simulink model "cic_filter_test_bitgrowthissue"  (Simulink 7.4)
settings: Solver=ode45  StartTime=0.0  StopTime=10000  RelTol=1e-3
libraries: xbsIndex_r4 x288, simulink x2, xrbsComm_r4 x1, xps_library x1
(part 2 of 3)

== system cic_filter_test_bitgrowthissue/myCIC/stage2 ==
  in1 : Inport
  in2 : Inport  Port=2
  sync : Inport  Port=3
  final_adder1 : xbsIndex_r4/AddSub  mode=Addition  use_carryin=off  use_carryout=off  en=off  latency=1  precision=Full  arith_type=Unsigned  n_bits=16  bin_pt=14  quantization=Truncate  overflow=Wrap  dbl_ovrd=off  use_behavioral_HDL=off  hw_selection=Fabric  pipelined=off  block_type=addsub
  polynomial0 : Subsystem
  polynomial1 : Subsystem
  sync_delay : xbsIndex_r4/Delay  en=off  latency=1  dbl_ovrd=off  reg_retiming=off  block_type=delay
      settings: block_version=11.4
  out1 : Outport
  sync_out : Outport  Port=2
  wires:
  sync/1 -> polynomial1/2(sync), polynomial0/2(sync)
  polynomial0/3(sync_out) -> sync_delay/1  "sync_poly"
  final_adder1/1 -> out1/1
  polynomial0/2(out_even) -> final_adder1/1  "poly_out0_even"
  in1/1 -> polynomial0/1(in)
  in2/1 -> polynomial1/1(in)
  polynomial1/1(out_odd) -> final_adder1/2  "poly_out1_odd"
  sync_delay/1 -> sync_out/1

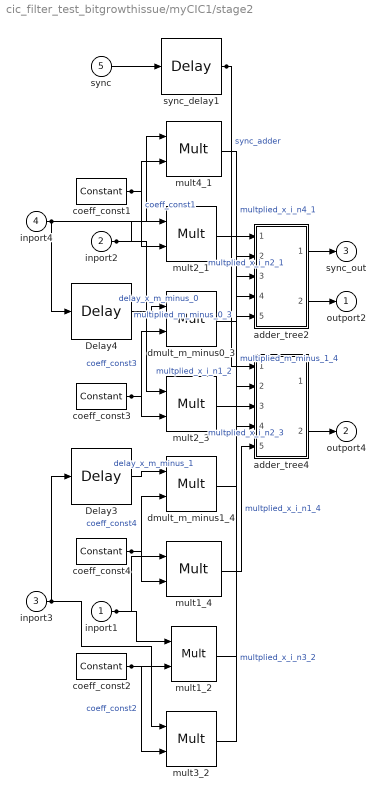
== system cic_filter_test_bitgrowthissue/myCIC1/stage2 ==
  inport1 : Inport
  inport2 : Inport  Port=2
  inport3 : Inport  Port=3
  inport4 : Inport  Port=4
  sync : Inport  Port=5
  Delay3 : xbsIndex_r4/Delay  en=off  latency=1  dbl_ovrd=off  reg_retiming=off  block_type=delay
      settings: block_version=11.4
  Delay4 : xbsIndex_r4/Delay  en=off  latency=1  dbl_ovrd=off  reg_retiming=off  block_type=delay
      settings: block_version=11.4
  adder_tree2 : Subsystem
  adder_tree4 : Subsystem
  coeff_const1 : xbsIndex_r4/Constant  arith_type=Unsigned  const=1  n_bits=3  bin_pt=0  explicit_period=off  period=1  equ=P=C  opselect=C  inp2=PCIN>>17  opr=+  inp1=P  carry=CIN  dbl_ovrd=off  block_type=constant
      settings: block_version=11.4
  coeff_const2 : xbsIndex_r4/Constant  arith_type=Unsigned  const=3  n_bits=3  bin_pt=0  explicit_period=off  period=1  equ=P=C  opselect=C  inp2=PCIN>>17  opr=+  inp1=P  carry=CIN  dbl_ovrd=off  block_type=constant
      settings: block_version=11.4
  coeff_const3 : xbsIndex_r4/Constant  arith_type=Unsigned  const=3  n_bits=3  bin_pt=0  explicit_period=off  period=1  equ=P=C  opselect=C  inp2=PCIN>>17  opr=+  inp1=P  carry=CIN  dbl_ovrd=off  block_type=constant
      settings: block_version=11.4
  coeff_const4 : xbsIndex_r4/Constant  arith_type=Unsigned  const=1  n_bits=3  bin_pt=0  explicit_period=off  period=1  equ=P=C  opselect=C  inp2=PCIN>>17  opr=+  inp1=P  carry=CIN  dbl_ovrd=off  block_type=constant
      settings: block_version=11.4
  dmult_m_minus0_3 : xbsIndex_r4/Mult  precision=Full  arith_type="Signed  (2's comp)"  n_bits=16  bin_pt=14  quantization=Truncate  overflow=Wrap  en=off  latency=2  dbl_ovrd=off  use_behavioral_HDL=off  opt=Speed  use_embedded=on  optimum_pipeline=off  pipeline=on  use_rpm=on  placement_style=Triangular  block_type=mult
      settings: block_version=11.4
  dmult_m_minus1_4 : xbsIndex_r4/Mult  precision=Full  arith_type="Signed  (2's comp)"  n_bits=16  bin_pt=14  quantization=Truncate  overflow=Wrap  en=off  latency=2  dbl_ovrd=off  use_behavioral_HDL=off  opt=Speed  use_embedded=on  optimum_pipeline=off  pipeline=on  use_rpm=on  placement_style=Triangular  block_type=mult
      settings: block_version=11.4
  mult1_2 : xbsIndex_r4/Mult  precision=Full  arith_type="Signed  (2's comp)"  n_bits=16  bin_pt=14  quantization=Truncate  overflow=Wrap  en=off  latency=2  dbl_ovrd=off  use_behavioral_HDL=off  opt=Speed  use_embedded=on  optimum_pipeline=off  pipeline=on  use_rpm=on  placement_style=Triangular  block_type=mult
      settings: block_version=11.4
  mult1_4 : xbsIndex_r4/Mult  precision=Full  arith_type="Signed  (2's comp)"  n_bits=16  bin_pt=14  quantization=Truncate  overflow=Wrap  en=off  latency=2  dbl_ovrd=off  use_behavioral_HDL=off  opt=Speed  use_embedded=on  optimum_pipeline=off  pipeline=on  use_rpm=on  placement_style=Triangular  block_type=mult
      settings: block_version=11.4
  mult2_1 : xbsIndex_r4/Mult  precision=Full  arith_type="Signed  (2's comp)"  n_bits=16  bin_pt=14  quantization=Truncate  overflow=Wrap  en=off  latency=2  dbl_ovrd=off  use_behavioral_HDL=off  opt=Speed  use_embedded=on  optimum_pipeline=off  pipeline=on  use_rpm=on  placement_style=Triangular  block_type=mult
      settings: block_version=11.4
  mult2_3 : xbsIndex_r4/Mult  precision=Full  arith_type="Signed  (2's comp)"  n_bits=16  bin_pt=14  quantization=Truncate  overflow=Wrap  en=off  latency=2  dbl_ovrd=off  use_behavioral_HDL=off  opt=Speed  use_embedded=on  optimum_pipeline=off  pipeline=on  use_rpm=on  placement_style=Triangular  block_type=mult
      settings: block_version=11.4
  mult3_2 : xbsIndex_r4/Mult  precision=Full  arith_type="Signed  (2's comp)"  n_bits=16  bin_pt=14  quantization=Truncate  overflow=Wrap  en=off  latency=2  dbl_ovrd=off  use_behavioral_HDL=off  opt=Speed  use_embedded=on  optimum_pipeline=off  pipeline=on  use_rpm=on  placement_style=Triangular  block_type=mult
      settings: block_version=11.4
  mult4_1 : xbsIndex_r4/Mult  precision=Full  arith_type="Signed  (2's comp)"  n_bits=16  bin_pt=14  quantization=Truncate  overflow=Wrap  en=off  latency=2  dbl_ovrd=off  use_behavioral_HDL=off  opt=Speed  use_embedded=on  optimum_pipeline=off  pipeline=on  use_rpm=on  placement_style=Triangular  block_type=mult
      settings: block_version=11.4
  sync_delay1 : xbsIndex_r4/Delay  en=off  latency=2  dbl_ovrd=off  reg_retiming=off  block_type=delay
      settings: block_version=11.4
  outport2 : Outport
  outport4 : Outport  Port=2
  sync_out : Outport  Port=3
  wires:
  inport1/1 -> mult1_2/1, mult1_4/1
  coeff_const4/1 -> mult1_4/2, dmult_m_minus1_4/2  "coeff_const4"
  inport2/1 -> mult2_1/1, mult2_3/1
  coeff_const3/1 -> mult2_3/2, dmult_m_minus0_3/2  "coeff_const3"
  inport3/1 -> mult3_2/1, Delay3/1
  coeff_const2/1 -> mult1_2/2, mult3_2/2  "coeff_const2"
  inport4/1 -> Delay4/1, mult4_1/1
  coeff_const1/1 -> mult4_1/2, mult2_1/2  "coeff_const1"
  sync_delay1/1 -> adder_tree4/1(sync), adder_tree2/1(sync)  "sync_adder"
  mult1_4/1 -> adder_tree4/5(din_4)  "multplied_x_i_n1_4"
  mult3_2/1 -> adder_tree4/3(din_2)  "multplied_x_i_n3_2"
  adder_tree2/2(dout) -> outport2/1
  dmult_m_minus1_4/1 -> adder_tree2/5(din_4)  "multiplied_m_minus_1_4"
  mult1_2/1 -> adder_tree2/3(din_2)  "multplied_x_i_n1_2"
  sync/1 -> sync_delay1/1
  Delay4/1 -> dmult_m_minus0_3/1  "delay_x_m_minus_0"
  Delay3/1 -> dmult_m_minus1_4/1  "delay_x_m_minus_1"
  mult2_1/1 -> adder_tree2/2(din_1)  "multplied_x_i_n2_1"
  dmult_m_minus0_3/1 -> adder_tree2/4(din_3)  "multiplied_m_minus_0_3"
  adder_tree2/1(sync_out) -> sync_out/1
  mult4_1/1 -> adder_tree4/2(din_1)  "multplied_x_i_n4_1"
  mult2_3/1 -> adder_tree4/4(din_3)  "multplied_x_i_n2_3"
  adder_tree4/2(dout) -> outport4/1

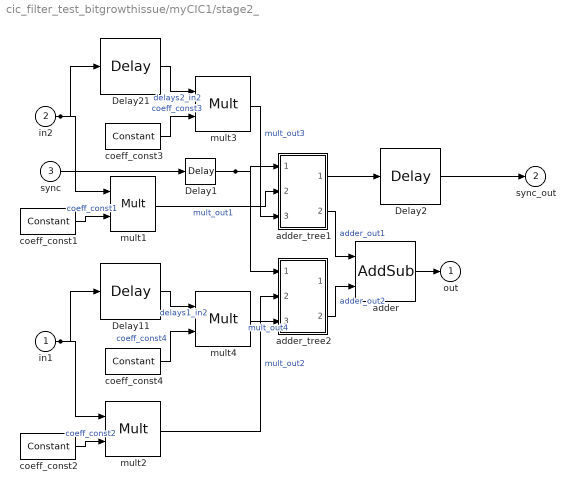
== system cic_filter_test_bitgrowthissue/myCIC1/stage2_ ==
  in1 : Inport
  in2 : Inport  Port=2
  sync : Inport  Port=3
  Delay1 : xbsIndex_r4/Delay  en=off  latency=2  dbl_ovrd=off  reg_retiming=off  block_type=delay
      settings: block_version=11.4
  Delay11 : xbsIndex_r4/Delay  en=off  latency=1  dbl_ovrd=off  reg_retiming=off  block_type=delay
      settings: block_version=11.4
  Delay2 : xbsIndex_r4/Delay  en=off  latency=1  dbl_ovrd=off  reg_retiming=off  block_type=delay
      settings: block_version=11.4
  Delay21 : xbsIndex_r4/Delay  en=off  latency=1  dbl_ovrd=off  reg_retiming=off  block_type=delay
      settings: block_version=11.4
  adder : xbsIndex_r4/AddSub  mode=Addition  use_carryin=off  use_carryout=off  en=off  latency=1  precision=Full  arith_type=Unsigned  n_bits=16  bin_pt=14  quantization=Truncate  overflow=Wrap  dbl_ovrd=off  use_behavioral_HDL=off  hw_selection=Fabric  pipelined=off  block_type=addsub
  adder_tree1 : Subsystem
  adder_tree2 : Subsystem
  coeff_const1 : xbsIndex_r4/Constant  arith_type=Unsigned  const=1  n_bits=3  bin_pt=0  explicit_period=off  period=1  equ=P=C  opselect=C  inp2=PCIN>>17  opr=+  inp1=P  carry=CIN  dbl_ovrd=off  block_type=constant
      settings: block_version=11.4
  coeff_const2 : xbsIndex_r4/Constant  arith_type=Unsigned  const=3  n_bits=3  bin_pt=0  explicit_period=off  period=1  equ=P=C  opselect=C  inp2=PCIN>>17  opr=+  inp1=P  carry=CIN  dbl_ovrd=off  block_type=constant
      settings: block_version=11.4
  coeff_const3 : xbsIndex_r4/Constant  arith_type=Unsigned  const=3  n_bits=3  bin_pt=0  explicit_period=off  period=1  equ=P=C  opselect=C  inp2=PCIN>>17  opr=+  inp1=P  carry=CIN  dbl_ovrd=off  block_type=constant
      settings: block_version=11.4
  coeff_const4 : xbsIndex_r4/Constant  arith_type=Unsigned  const=1  n_bits=3  bin_pt=0  explicit_period=off  period=1  equ=P=C  opselect=C  inp2=PCIN>>17  opr=+  inp1=P  carry=CIN  dbl_ovrd=off  block_type=constant
      settings: block_version=11.4
  mult{1..4} (4 alike) : xbsIndex_r4/Mult  precision=Full  arith_type="Signed  (2's comp)"  n_bits=16  bin_pt=14  quantization=Truncate  overflow=Wrap  en=off  latency=2  dbl_ovrd=off  use_behavioral_HDL=off  opt=Speed  use_embedded=on  optimum_pipeline=off  pipeline=on  use_rpm=on  placement_style=Triangular  block_type=mult
      settings: block_version=11.4
  out : Outport
  sync_out : Outport  Port=2
  wires:
  in2/1 -> mult1/1, Delay21/1
  in1/1 -> Delay11/1, mult2/1
  sync/1 -> Delay1/1
  adder_tree2/2(dout) -> adder/2  "adder_out2"
  mult2/1 -> adder_tree2/2(din_1)  "mult_out2"
  mult3/1 -> adder_tree1/3(din_2)  "mult_out3"
  coeff_const4/1 -> mult4/2  "coeff_const4"
  Delay21/1 -> mult3/1  "delays2_in2"
  coeff_const2/1 -> mult2/2  "coeff_const2"
  coeff_const1/1 -> mult1/2  "coeff_const1"
  coeff_const3/1 -> mult3/2  "coeff_const3"
  Delay11/1 -> mult4/1  "delays1_in2"
  mult1/1 -> adder_tree1/2(din_1)  "mult_out1"
  adder_tree1/1(sync_out) -> Delay2/1
  mult4/1 -> adder_tree2/3(din_2)  "mult_out4"
  adder_tree1/2(dout) -> adder/1  "adder_out1"
  adder/1 -> out/1
  Delay1/1 -> adder_tree1/1(sync), adder_tree2/1(sync)
  Delay2/1 -> sync_out/1

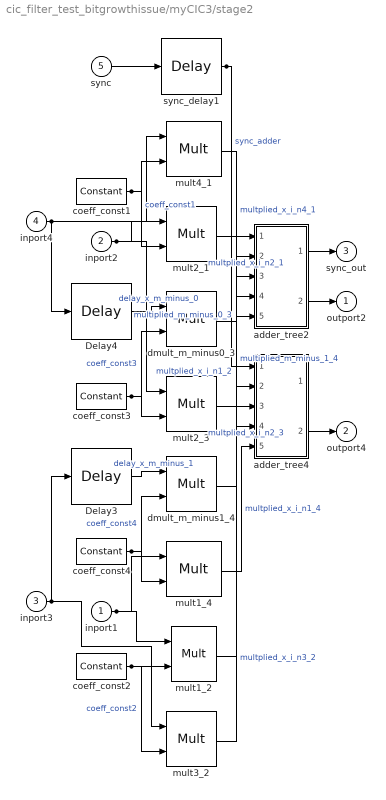
== system cic_filter_test_bitgrowthissue/myCIC3/stage2 ==
  inport1 : Inport
  inport2 : Inport  Port=2
  inport3 : Inport  Port=3
  inport4 : Inport  Port=4
  sync : Inport  Port=5
  Delay3 : xbsIndex_r4/Delay  en=off  latency=1  dbl_ovrd=off  reg_retiming=off  block_type=delay
      settings: block_version=11.4
  Delay4 : xbsIndex_r4/Delay  en=off  latency=1  dbl_ovrd=off  reg_retiming=off  block_type=delay
      settings: block_version=11.4
  adder_tree2 : Subsystem
  adder_tree4 : Subsystem
  coeff_const1 : xbsIndex_r4/Constant  arith_type=Unsigned  const=1  n_bits=3  bin_pt=0  explicit_period=off  period=1  equ=P=C  opselect=C  inp2=PCIN>>17  opr=+  inp1=P  carry=CIN  dbl_ovrd=off  block_type=constant
      settings: block_version=11.4
  coeff_const2 : xbsIndex_r4/Constant  arith_type=Unsigned  const=3  n_bits=3  bin_pt=0  explicit_period=off  period=1  equ=P=C  opselect=C  inp2=PCIN>>17  opr=+  inp1=P  carry=CIN  dbl_ovrd=off  block_type=constant
      settings: block_version=11.4
  coeff_const3 : xbsIndex_r4/Constant  arith_type=Unsigned  const=3  n_bits=3  bin_pt=0  explicit_period=off  period=1  equ=P=C  opselect=C  inp2=PCIN>>17  opr=+  inp1=P  carry=CIN  dbl_ovrd=off  block_type=constant
      settings: block_version=11.4
  coeff_const4 : xbsIndex_r4/Constant  arith_type=Unsigned  const=1  n_bits=3  bin_pt=0  explicit_period=off  period=1  equ=P=C  opselect=C  inp2=PCIN>>17  opr=+  inp1=P  carry=CIN  dbl_ovrd=off  block_type=constant
      settings: block_version=11.4
  dmult_m_minus0_3 : xbsIndex_r4/Mult  precision=Full  arith_type="Signed  (2's comp)"  n_bits=16  bin_pt=14  quantization=Truncate  overflow=Wrap  en=off  latency=2  dbl_ovrd=off  use_behavioral_HDL=off  opt=Speed  use_embedded=on  optimum_pipeline=off  pipeline=on  use_rpm=on  placement_style=Triangular  block_type=mult
      settings: block_version=11.4
  dmult_m_minus1_4 : xbsIndex_r4/Mult  precision=Full  arith_type="Signed  (2's comp)"  n_bits=16  bin_pt=14  quantization=Truncate  overflow=Wrap  en=off  latency=2  dbl_ovrd=off  use_behavioral_HDL=off  opt=Speed  use_embedded=on  optimum_pipeline=off  pipeline=on  use_rpm=on  placement_style=Triangular  block_type=mult
      settings: block_version=11.4
  mult1_2 : xbsIndex_r4/Mult  precision=Full  arith_type="Signed  (2's comp)"  n_bits=16  bin_pt=14  quantization=Truncate  overflow=Wrap  en=off  latency=2  dbl_ovrd=off  use_behavioral_HDL=off  opt=Speed  use_embedded=on  optimum_pipeline=off  pipeline=on  use_rpm=on  placement_style=Triangular  block_type=mult
      settings: block_version=11.4
  mult1_4 : xbsIndex_r4/Mult  precision=Full  arith_type="Signed  (2's comp)"  n_bits=16  bin_pt=14  quantization=Truncate  overflow=Wrap  en=off  latency=2  dbl_ovrd=off  use_behavioral_HDL=off  opt=Speed  use_embedded=on  optimum_pipeline=off  pipeline=on  use_rpm=on  placement_style=Triangular  block_type=mult
      settings: block_version=11.4
  mult2_1 : xbsIndex_r4/Mult  precision=Full  arith_type="Signed  (2's comp)"  n_bits=16  bin_pt=14  quantization=Truncate  overflow=Wrap  en=off  latency=2  dbl_ovrd=off  use_behavioral_HDL=off  opt=Speed  use_embedded=on  optimum_pipeline=off  pipeline=on  use_rpm=on  placement_style=Triangular  block_type=mult
      settings: block_version=11.4
  mult2_3 : xbsIndex_r4/Mult  precision=Full  arith_type="Signed  (2's comp)"  n_bits=16  bin_pt=14  quantization=Truncate  overflow=Wrap  en=off  latency=2  dbl_ovrd=off  use_behavioral_HDL=off  opt=Speed  use_embedded=on  optimum_pipeline=off  pipeline=on  use_rpm=on  placement_style=Triangular  block_type=mult
      settings: block_version=11.4
  mult3_2 : xbsIndex_r4/Mult  precision=Full  arith_type="Signed  (2's comp)"  n_bits=16  bin_pt=14  quantization=Truncate  overflow=Wrap  en=off  latency=2  dbl_ovrd=off  use_behavioral_HDL=off  opt=Speed  use_embedded=on  optimum_pipeline=off  pipeline=on  use_rpm=on  placement_style=Triangular  block_type=mult
      settings: block_version=11.4
  mult4_1 : xbsIndex_r4/Mult  precision=Full  arith_type="Signed  (2's comp)"  n_bits=16  bin_pt=14  quantization=Truncate  overflow=Wrap  en=off  latency=2  dbl_ovrd=off  use_behavioral_HDL=off  opt=Speed  use_embedded=on  optimum_pipeline=off  pipeline=on  use_rpm=on  placement_style=Triangular  block_type=mult
      settings: block_version=11.4
  sync_delay1 : xbsIndex_r4/Delay  en=off  latency=2  dbl_ovrd=off  reg_retiming=off  block_type=delay
      settings: block_version=11.4
  outport2 : Outport
  outport4 : Outport  Port=2
  sync_out : Outport  Port=3
  wires:
  inport1/1 -> mult1_2/1, mult1_4/1
  coeff_const4/1 -> mult1_4/2, dmult_m_minus1_4/2  "coeff_const4"
  inport2/1 -> mult2_1/1, mult2_3/1
  coeff_const3/1 -> mult2_3/2, dmult_m_minus0_3/2  "coeff_const3"
  inport3/1 -> mult3_2/1, Delay3/1
  coeff_const2/1 -> mult1_2/2, mult3_2/2  "coeff_const2"
  inport4/1 -> Delay4/1, mult4_1/1
  coeff_const1/1 -> mult4_1/2, mult2_1/2  "coeff_const1"
  sync_delay1/1 -> adder_tree4/1(sync), adder_tree2/1(sync)  "sync_adder"
  mult1_4/1 -> adder_tree4/5(din_4)  "multplied_x_i_n1_4"
  mult3_2/1 -> adder_tree4/3(din_2)  "multplied_x_i_n3_2"
  adder_tree2/2(dout) -> outport2/1
  dmult_m_minus1_4/1 -> adder_tree2/5(din_4)  "multiplied_m_minus_1_4"
  mult1_2/1 -> adder_tree2/3(din_2)  "multplied_x_i_n1_2"
  sync/1 -> sync_delay1/1
  Delay4/1 -> dmult_m_minus0_3/1  "delay_x_m_minus_0"
  Delay3/1 -> dmult_m_minus1_4/1  "delay_x_m_minus_1"
  mult2_1/1 -> adder_tree2/2(din_1)  "multplied_x_i_n2_1"
  dmult_m_minus0_3/1 -> adder_tree2/4(din_3)  "multiplied_m_minus_0_3"
  adder_tree2/1(sync_out) -> sync_out/1
  mult4_1/1 -> adder_tree4/2(din_1)  "multplied_x_i_n4_1"
  mult2_3/1 -> adder_tree4/4(din_3)  "multplied_x_i_n2_3"
  adder_tree4/2(dout) -> outport4/1

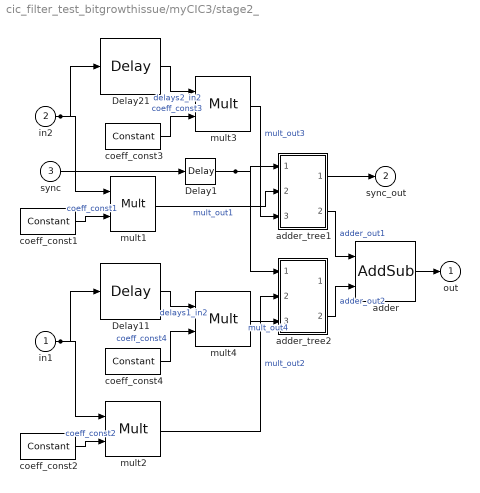
== system cic_filter_test_bitgrowthissue/myCIC3/stage2_ ==
  in1 : Inport
  in2 : Inport  Port=2
  sync : Inport  Port=3
  Delay1 : xbsIndex_r4/Delay  en=off  latency=2  dbl_ovrd=off  reg_retiming=off  block_type=delay
      settings: block_version=11.4
  Delay11 : xbsIndex_r4/Delay  en=off  latency=1  dbl_ovrd=off  reg_retiming=off  block_type=delay
      settings: block_version=11.4
  Delay21 : xbsIndex_r4/Delay  en=off  latency=1  dbl_ovrd=off  reg_retiming=off  block_type=delay
      settings: block_version=11.4
  adder : xbsIndex_r4/AddSub  mode=Addition  use_carryin=off  use_carryout=off  en=off  latency=1  precision=Full  arith_type=Unsigned  n_bits=16  bin_pt=14  quantization=Truncate  overflow=Wrap  dbl_ovrd=off  use_behavioral_HDL=off  hw_selection=Fabric  pipelined=off  block_type=addsub
  adder_tree1 : Subsystem
  adder_tree2 : Subsystem
  coeff_const1 : xbsIndex_r4/Constant  arith_type=Unsigned  const=1  n_bits=3  bin_pt=0  explicit_period=off  period=1  equ=P=C  opselect=C  inp2=PCIN>>17  opr=+  inp1=P  carry=CIN  dbl_ovrd=off  block_type=constant
      settings: block_version=11.4
  coeff_const2 : xbsIndex_r4/Constant  arith_type=Unsigned  const=3  n_bits=3  bin_pt=0  explicit_period=off  period=1  equ=P=C  opselect=C  inp2=PCIN>>17  opr=+  inp1=P  carry=CIN  dbl_ovrd=off  block_type=constant
      settings: block_version=11.4
  coeff_const3 : xbsIndex_r4/Constant  arith_type=Unsigned  const=3  n_bits=3  bin_pt=0  explicit_period=off  period=1  equ=P=C  opselect=C  inp2=PCIN>>17  opr=+  inp1=P  carry=CIN  dbl_ovrd=off  block_type=constant
      settings: block_version=11.4
  coeff_const4 : xbsIndex_r4/Constant  arith_type=Unsigned  const=1  n_bits=3  bin_pt=0  explicit_period=off  period=1  equ=P=C  opselect=C  inp2=PCIN>>17  opr=+  inp1=P  carry=CIN  dbl_ovrd=off  block_type=constant
      settings: block_version=11.4
  mult{1..4} (4 alike) : xbsIndex_r4/Mult  precision=Full  arith_type="Signed  (2's comp)"  n_bits=16  bin_pt=14  quantization=Truncate  overflow=Wrap  en=off  latency=2  dbl_ovrd=off  use_behavioral_HDL=off  opt=Speed  use_embedded=on  optimum_pipeline=off  pipeline=on  use_rpm=on  placement_style=Triangular  block_type=mult
      settings: block_version=11.4
  out : Outport
  sync_out : Outport  Port=2
  wires:
  in2/1 -> mult1/1, Delay21/1
  in1/1 -> Delay11/1, mult2/1
  sync/1 -> Delay1/1
  adder_tree2/2(dout) -> adder/2  "adder_out2"
  mult2/1 -> adder_tree2/2(din_1)  "mult_out2"
  mult3/1 -> adder_tree1/3(din_2)  "mult_out3"
  coeff_const4/1 -> mult4/2  "coeff_const4"
  Delay21/1 -> mult3/1  "delays2_in2"
  coeff_const2/1 -> mult2/2  "coeff_const2"
  coeff_const1/1 -> mult1/2  "coeff_const1"
  coeff_const3/1 -> mult3/2  "coeff_const3"
  Delay11/1 -> mult4/1  "delays1_in2"
  mult1/1 -> adder_tree1/2(din_1)  "mult_out1"
  adder_tree1/1(sync_out) -> sync_out/1
  mult4/1 -> adder_tree2/3(din_2)  "mult_out4"
  adder_tree1/2(dout) -> adder/1  "adder_out1"
  adder/1 -> out/1
  Delay1/1 -> adder_tree1/1(sync), adder_tree2/1(sync)

== system cic_filter_test_bitgrowthissue/non parallel CIC/stage1 ==
  inport : Inport
  sync : Inport  Port=2
  Down_sample0 : xbsIndex_r4/Down Sample  sample_ratio=2  sample_phase="Last Value of Frame  (most efficient)"  en=off  latency=1  dbl_ovrd=off  block_type=dsamp
      settings: block_version=11.4
  Down_sample1 : xbsIndex_r4/Down Sample  sample_ratio=2  sample_phase="Last Value of Frame  (most efficient)"  en=off  latency=1  dbl_ovrd=off  block_type=dsamp
      settings: block_version=11.4
  final_adder : xbsIndex_r4/AddSub  mode=Addition  use_carryin=off  use_carryout=off  en=off  latency=1  precision=Full  arith_type=Unsigned  n_bits=16  bin_pt=14  quantization=Truncate  overflow=Wrap  dbl_ovrd=off  use_behavioral_HDL=off  hw_selection=Fabric  pipelined=off  block_type=addsub
  first_delay : xbsIndex_r4/Delay  en=off  latency=1  dbl_ovrd=off  reg_retiming=off  block_type=delay
      settings: block_version=11.4
  polynomial0 : Subsystem
  polynomial1 : Subsystem
  sync_delay : xbsIndex_r4/Delay  en=off  latency=2  dbl_ovrd=off  reg_retiming=off  block_type=delay
      settings: block_version=11.4
  outport : Outport
  sync_out : Outport  Port=2
  wires:
  inport/1 -> Down_sample0/1, first_delay/1
  sync/1 -> polynomial1/2(sync), polynomial0/2(sync)
  polynomial0/2(sync_out) -> sync_delay/1  "sync_poly"
  final_adder/1 -> outport/1
  polynomial0/1(out) -> final_adder/1  "poly_out0"
  Down_sample0/1 -> polynomial0/1(in)  "downsample_out0"
  first_delay/1 -> Down_sample1/1  "delay1"
  Down_sample1/1 -> polynomial1/1(in)  "downsample_out1"
  polynomial1/1(out) -> final_adder/2  "poly_out1"
  sync_delay/1 -> sync_out/1

== system cic_filter_test_bitgrowthissue/non parallel CIC/stage2 ==
  inport : Inport
  sync : Inport  Port=2
  Down_sample0 : xbsIndex_r4/Down Sample  sample_ratio=2  sample_phase="Last Value of Frame  (most efficient)"  en=off  latency=1  dbl_ovrd=off  block_type=dsamp
      settings: block_version=11.4
  Down_sample1 : xbsIndex_r4/Down Sample  sample_ratio=2  sample_phase="Last Value of Frame  (most efficient)"  en=off  latency=1  dbl_ovrd=off  block_type=dsamp
      settings: block_version=11.4
  final_adder : xbsIndex_r4/AddSub  mode=Addition  use_carryin=off  use_carryout=off  en=off  latency=1  precision=Full  arith_type=Unsigned  n_bits=16  bin_pt=14  quantization=Truncate  overflow=Wrap  dbl_ovrd=off  use_behavioral_HDL=off  hw_selection=Fabric  pipelined=off  block_type=addsub
  first_delay : xbsIndex_r4/Delay  en=off  latency=1  dbl_ovrd=off  reg_retiming=off  block_type=delay
      settings: block_version=11.4
  polynomial0 : Subsystem
  polynomial1 : Subsystem
  sync_delay : xbsIndex_r4/Delay  en=off  latency=2  dbl_ovrd=off  reg_retiming=off  block_type=delay
      settings: block_version=11.4
  outport : Outport
  sync_out : Outport  Port=2
  wires:
  inport/1 -> Down_sample0/1, first_delay/1
  sync/1 -> polynomial1/2(sync), polynomial0/2(sync)
  polynomial0/2(sync_out) -> sync_delay/1  "sync_poly"
  final_adder/1 -> outport/1
  polynomial0/1(out) -> final_adder/1  "poly_out0"
  Down_sample0/1 -> polynomial0/1(in)  "downsample_out0"
  first_delay/1 -> Down_sample1/1  "delay1"
  Down_sample1/1 -> polynomial1/1(in)  "downsample_out1"
  polynomial1/1(out) -> final_adder/2  "poly_out1"
  sync_delay/1 -> sync_out/1

== system cic_filter_test_bitgrowthissue/non parallel CIC/stage3 ==
  inport : Inport
  sync : Inport  Port=2
  Down_sample0 : xbsIndex_r4/Down Sample  sample_ratio=2  sample_phase="Last Value of Frame  (most efficient)"  en=off  latency=1  dbl_ovrd=off  block_type=dsamp
      settings: block_version=11.4
  Down_sample1 : xbsIndex_r4/Down Sample  sample_ratio=2  sample_phase="Last Value of Frame  (most efficient)"  en=off  latency=1  dbl_ovrd=off  block_type=dsamp
      settings: block_version=11.4
  final_adder : xbsIndex_r4/AddSub  mode=Addition  use_carryin=off  use_carryout=off  en=off  latency=1  precision=Full  arith_type=Unsigned  n_bits=16  bin_pt=14  quantization=Truncate  overflow=Wrap  dbl_ovrd=off  use_behavioral_HDL=off  hw_selection=Fabric  pipelined=off  block_type=addsub
  first_delay : xbsIndex_r4/Delay  en=off  latency=1  dbl_ovrd=off  reg_retiming=off  block_type=delay
      settings: block_version=11.4
  polynomial0 : Subsystem
  polynomial1 : Subsystem
  sync_delay : xbsIndex_r4/Delay  en=off  latency=2  dbl_ovrd=off  reg_retiming=off  block_type=delay
      settings: block_version=11.4
  outport : Outport
  sync_out : Outport  Port=2
  wires:
  inport/1 -> Down_sample0/1, first_delay/1
  sync/1 -> polynomial1/2(sync), polynomial0/2(sync)
  polynomial0/2(sync_out) -> sync_delay/1  "sync_poly"
  final_adder/1 -> outport/1
  polynomial0/1(out) -> final_adder/1  "poly_out0"
  Down_sample0/1 -> polynomial0/1(in)  "downsample_out0"
  first_delay/1 -> Down_sample1/1  "delay1"
  Down_sample1/1 -> polynomial1/1(in)  "downsample_out1"
  polynomial1/1(out) -> final_adder/2  "poly_out1"
  sync_delay/1 -> sync_out/1

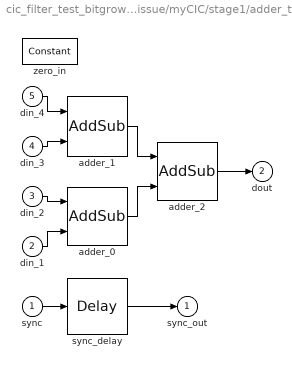
== system cic_filter_test_bitgrowthissue/myCIC/stage1/adder_tree1 ==
  sync : Inport
  din_1 : Inport  Port=2
  din_2 : Inport  Port=3
  din_3 : Inport  Port=4
  din_4 : Inport  Port=5
  adder_0 : xbsIndex_r4/AddSub  mode=Addition  use_carryin=off  use_carryout=off  en=off  latency=1  precision=Full  arith_type=Unsigned  n_bits=16  bin_pt=14  quantization="Round  (unbiased: +/- Inf)"  overflow=Saturate  dbl_ovrd=off  use_behavioral_HDL=on  hw_selection=Fabric  pipelined=off  block_type=addsub
  adder_1 : xbsIndex_r4/AddSub  mode=Addition  use_carryin=off  use_carryout=off  en=off  latency=1  precision=Full  arith_type=Unsigned  n_bits=16  bin_pt=14  quantization="Round  (unbiased: +/- Inf)"  overflow=Saturate  dbl_ovrd=off  use_behavioral_HDL=on  hw_selection=Fabric  pipelined=off  block_type=addsub
  adder_2 : xbsIndex_r4/AddSub  mode=Addition  use_carryin=off  use_carryout=off  en=off  latency=1  precision=Full  arith_type=Unsigned  n_bits=16  bin_pt=14  quantization="Round  (unbiased: +/- Inf)"  overflow=Saturate  dbl_ovrd=off  use_behavioral_HDL=on  hw_selection=Fabric  pipelined=off  block_type=addsub
  sync_delay : xbsIndex_r4/Delay  en=off  latency=2  dbl_ovrd=off  reg_retiming=off  block_type=delay
      settings: block_version=11.4
  zero_in : xbsIndex_r4/Constant  arith_type=Unsigned  const=0  n_bits=18  bin_pt=17  explicit_period=off  period=1  equ=P=C  opselect=C  inp2=PCIN>>17  opr=+  inp1=P  carry=CIN  dbl_ovrd=off  block_type=constant
      settings: block_version=11.4
  sync_out : Outport
  dout : Outport  Port=2
  wires:
  adder_0/1 -> adder_2/2
  din_4/1 -> adder_1/1
  din_1/1 -> adder_0/2
  sync_delay/1 -> sync_out/1
  sync/1 -> sync_delay/1
  din_2/1 -> adder_0/1
  din_3/1 -> adder_1/2
  adder_1/1 -> adder_2/1
  adder_2/1 -> dout/1

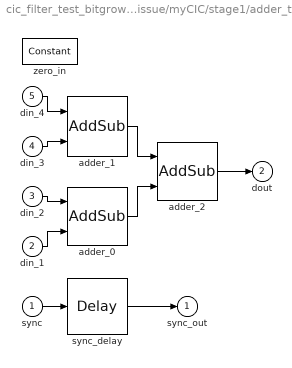
== system cic_filter_test_bitgrowthissue/myCIC/stage1/adder_tree3 ==
  sync : Inport
  din_1 : Inport  Port=2
  din_2 : Inport  Port=3
  din_3 : Inport  Port=4
  din_4 : Inport  Port=5
  adder_0 : xbsIndex_r4/AddSub  mode=Addition  use_carryin=off  use_carryout=off  en=off  latency=1  precision=Full  arith_type=Unsigned  n_bits=16  bin_pt=14  quantization="Round  (unbiased: +/- Inf)"  overflow=Saturate  dbl_ovrd=off  use_behavioral_HDL=on  hw_selection=Fabric  pipelined=off  block_type=addsub
  adder_1 : xbsIndex_r4/AddSub  mode=Addition  use_carryin=off  use_carryout=off  en=off  latency=1  precision=Full  arith_type=Unsigned  n_bits=16  bin_pt=14  quantization="Round  (unbiased: +/- Inf)"  overflow=Saturate  dbl_ovrd=off  use_behavioral_HDL=on  hw_selection=Fabric  pipelined=off  block_type=addsub
  adder_2 : xbsIndex_r4/AddSub  mode=Addition  use_carryin=off  use_carryout=off  en=off  latency=1  precision=Full  arith_type=Unsigned  n_bits=16  bin_pt=14  quantization="Round  (unbiased: +/- Inf)"  overflow=Saturate  dbl_ovrd=off  use_behavioral_HDL=on  hw_selection=Fabric  pipelined=off  block_type=addsub
  sync_delay : xbsIndex_r4/Delay  en=off  latency=2  dbl_ovrd=off  reg_retiming=off  block_type=delay
      settings: block_version=11.4
  zero_in : xbsIndex_r4/Constant  arith_type=Unsigned  const=0  n_bits=18  bin_pt=17  explicit_period=off  period=1  equ=P=C  opselect=C  inp2=PCIN>>17  opr=+  inp1=P  carry=CIN  dbl_ovrd=off  block_type=constant
      settings: block_version=11.4
  sync_out : Outport
  dout : Outport  Port=2
  wires:
  adder_0/1 -> adder_2/2
  din_4/1 -> adder_1/1
  din_1/1 -> adder_0/2
  sync_delay/1 -> sync_out/1
  sync/1 -> sync_delay/1
  din_2/1 -> adder_0/1
  din_3/1 -> adder_1/2
  adder_1/1 -> adder_2/1
  adder_2/1 -> dout/1

== system cic_filter_test_bitgrowthissue/myCIC/stage1/mult_cxi_blk1 ==
  in : Inport
  sync : Inport  Port=2
  adder_tree2 : Subsystem
  delay1 : xbsIndex_r4/Delay  en=off  latency=1  dbl_ovrd=off  reg_retiming=off  block_type=delay
      settings: block_version=11.4
  shift2 : xbsIndex_r4/Shift  shift_dir=Left  shift_bits=1  en=off  latency=0  precision=Full  arith_type="Signed  (2's comp)"  n_bits=16  bin_pt=14  quantization=Truncate  overflow=Wrap  dbl_ovrd=off  block_type=shift
  sync_delay : xbsIndex_r4/Delay  en=off  latency=1  dbl_ovrd=off  reg_retiming=off  block_type=delay
      settings: block_version=11.4
  out1 : Outport
  out2 : Outport  Port=2
  sync_out : Outport  Port=3
  wires:
  in/1 -> delay1/1, adder_tree2/1(sync), shift2/1, adder_tree2/2(din_1)  "adder_trees_out1"
  sync/1 -> sync_delay/1
  delay1/1 -> out1/1  "out1"
  shift2/1 -> adder_tree2/3(din_2)  "shift_out2"
  adder_tree2/2(dout) -> out2/1  "out2"
  sync_delay/1 -> sync_out/1

== system cic_filter_test_bitgrowthissue/myCIC/stage1/mult_cxi_blk2 ==
  in : Inport
  sync : Inport  Port=2
  adder_tree1 : Subsystem
  delay2 : xbsIndex_r4/Delay  en=off  latency=1  dbl_ovrd=off  reg_retiming=off  block_type=delay
      settings: block_version=11.4
  shift2 : xbsIndex_r4/Shift  shift_dir=Left  shift_bits=1  en=off  latency=0  precision=Full  arith_type="Signed  (2's comp)"  n_bits=16  bin_pt=14  quantization=Truncate  overflow=Wrap  dbl_ovrd=off  block_type=shift
  sync_delay : xbsIndex_r4/Delay  en=off  latency=1  dbl_ovrd=off  reg_retiming=off  block_type=delay
      settings: block_version=11.4
  out1 : Outport
  out2 : Outport  Port=2
  sync_out : Outport  Port=3
  wires:
  in/1 -> delay2/1, adder_tree1/1(sync), shift2/1, adder_tree1/2(din_1)  "adder_trees_out2"
  sync/1 -> sync_delay/1
  adder_tree1/2(dout) -> out1/1  "out1"
  shift2/1 -> adder_tree1/3(din_2)  "shift_out2"
  delay2/1 -> out2/1  "out2"
  sync_delay/1 -> sync_out/1

== system cic_filter_test_bitgrowthissue/myCIC/stage1/mult_cxi_blk3 ==
  in : Inport
  sync : Inport  Port=2
  adder_tree2 : Subsystem
  delay1 : xbsIndex_r4/Delay  en=off  latency=1  dbl_ovrd=off  reg_retiming=off  block_type=delay
      settings: block_version=11.4
  shift2 : xbsIndex_r4/Shift  shift_dir=Left  shift_bits=1  en=off  latency=0  precision=Full  arith_type="Signed  (2's comp)"  n_bits=16  bin_pt=14  quantization=Truncate  overflow=Wrap  dbl_ovrd=off  block_type=shift
  sync_delay : xbsIndex_r4/Delay  en=off  latency=1  dbl_ovrd=off  reg_retiming=off  block_type=delay
      settings: block_version=11.4
  out1 : Outport
  out2 : Outport  Port=2
  sync_out : Outport  Port=3
  wires:
  in/1 -> delay1/1, adder_tree2/1(sync), shift2/1, adder_tree2/2(din_1)  "adder_trees_out1"
  sync/1 -> sync_delay/1
  delay1/1 -> out1/1  "out1"
  shift2/1 -> adder_tree2/3(din_2)  "shift_out2"
  adder_tree2/2(dout) -> out2/1  "out2"
  sync_delay/1 -> sync_out/1

== system cic_filter_test_bitgrowthissue/myCIC/stage1/mult_cxi_blk4 ==
  in : Inport
  sync : Inport  Port=2
  adder_tree1 : Subsystem
  delay2 : xbsIndex_r4/Delay  en=off  latency=1  dbl_ovrd=off  reg_retiming=off  block_type=delay
      settings: block_version=11.4
  shift2 : xbsIndex_r4/Shift  shift_dir=Left  shift_bits=1  en=off  latency=0  precision=Full  arith_type="Signed  (2's comp)"  n_bits=16  bin_pt=14  quantization=Truncate  overflow=Wrap  dbl_ovrd=off  block_type=shift
  sync_delay : xbsIndex_r4/Delay  en=off  latency=1  dbl_ovrd=off  reg_retiming=off  block_type=delay
      settings: block_version=11.4
  out1 : Outport
  out2 : Outport  Port=2
  sync_out : Outport  Port=3
  wires:
  in/1 -> delay2/1, adder_tree1/1(sync), shift2/1, adder_tree1/2(din_1)  "adder_trees_out2"
  sync/1 -> sync_delay/1
  adder_tree1/2(dout) -> out1/1  "out1"
  shift2/1 -> adder_tree1/3(din_2)  "shift_out2"
  delay2/1 -> out2/1  "out2"
  sync_delay/1 -> sync_out/1

== system cic_filter_test_bitgrowthissue/myCIC/stage2/polynomial0 ==
  in : Inport
  sync : Inport  Port=2
  even_adder_blk1 : xbsIndex_r4/AddSub  mode=Addition  use_carryin=off  use_carryout=off  en=off  latency=1  precision=Full  arith_type=Unsigned  n_bits=16  bin_pt=14  quantization=Truncate  overflow=Wrap  dbl_ovrd=off  use_behavioral_HDL=off  hw_selection=Fabric  pipelined=off  block_type=addsub
  even_delay1 : xbsIndex_r4/Delay  en=off  latency=1  dbl_ovrd=off  reg_retiming=off  block_type=delay
      settings: block_version=11.4
  odd_adder_blk1 : xbsIndex_r4/AddSub  mode=Addition  use_carryin=off  use_carryout=off  en=off  latency=1  precision=Full  arith_type=Unsigned  n_bits=16  bin_pt=14  quantization=Truncate  overflow=Wrap  dbl_ovrd=off  use_behavioral_HDL=off  hw_selection=Fabric  pipelined=off  block_type=addsub
  odd_delay1 : xbsIndex_r4/Delay  en=off  latency=1  dbl_ovrd=off  reg_retiming=off  block_type=delay
      settings: block_version=11.4
  shift_mult_array : Subsystem
  sync_delay1 : xbsIndex_r4/Delay  en=off  latency=1  dbl_ovrd=off  reg_retiming=off  block_type=delay
      settings: block_version=11.4
  out_odd : Outport
  out_even : Outport  Port=2
  sync_out : Outport  Port=3
  wires:
  shift_mult_array/5(sync_out) -> sync_delay1/1  "sync_mult"
  odd_adder_blk1/1 -> out_odd/1  "odd_delay_in2"
  shift_mult_array/2(out2) -> even_adder_blk1/2  "mult_out2"
  odd_delay1/1 -> odd_adder_blk1/1  "odd_delay_out1"
  shift_mult_array/3(out3) -> odd_delay1/1  "mult_out3"
  sync/1 -> shift_mult_array/2(sync)
  in/1 -> shift_mult_array/1(in)
  shift_mult_array/1(out1) -> odd_adder_blk1/2  "mult_out1"
  shift_mult_array/4(out4) -> even_delay1/1  "mult_out4"
  even_delay1/1 -> even_adder_blk1/1  "even_delay_out1"
  even_adder_blk1/1 -> out_even/1  "even_delay_in2"
  sync_delay1/1 -> sync_out/1

== system cic_filter_test_bitgrowthissue/myCIC/stage2/polynomial1 ==
  in : Inport
  sync : Inport  Port=2
  even_adder_blk1 : xbsIndex_r4/AddSub  mode=Addition  use_carryin=off  use_carryout=off  en=off  latency=1  precision=Full  arith_type=Unsigned  n_bits=16  bin_pt=14  quantization=Truncate  overflow=Wrap  dbl_ovrd=off  use_behavioral_HDL=off  hw_selection=Fabric  pipelined=off  block_type=addsub
  even_delay1 : xbsIndex_r4/Delay  en=off  latency=1  dbl_ovrd=off  reg_retiming=off  block_type=delay
      settings: block_version=11.4
  odd_adder_blk1 : xbsIndex_r4/AddSub  mode=Addition  use_carryin=off  use_carryout=off  en=off  latency=1  precision=Full  arith_type=Unsigned  n_bits=16  bin_pt=14  quantization=Truncate  overflow=Wrap  dbl_ovrd=off  use_behavioral_HDL=off  hw_selection=Fabric  pipelined=off  block_type=addsub
  odd_delay1 : xbsIndex_r4/Delay  en=off  latency=1  dbl_ovrd=off  reg_retiming=off  block_type=delay
      settings: block_version=11.4
  shift_mult_array : Subsystem
  sync_delay1 : xbsIndex_r4/Delay  en=off  latency=1  dbl_ovrd=off  reg_retiming=off  block_type=delay
      settings: block_version=11.4
  out_odd : Outport
  out_even : Outport  Port=2
  sync_out : Outport  Port=3
  wires:
  shift_mult_array/5(sync_out) -> sync_delay1/1  "sync_mult"
  odd_adder_blk1/1 -> out_odd/1  "odd_delay_in2"
  shift_mult_array/2(out2) -> even_adder_blk1/2  "mult_out2"
  odd_delay1/1 -> odd_adder_blk1/1  "odd_delay_out1"
  shift_mult_array/3(out3) -> odd_delay1/1  "mult_out3"
  sync/1 -> shift_mult_array/2(sync)
  in/1 -> shift_mult_array/1(in)
  shift_mult_array/1(out1) -> odd_adder_blk1/2  "mult_out1"
  shift_mult_array/4(out4) -> even_delay1/1  "mult_out4"
  even_delay1/1 -> even_adder_blk1/1  "even_delay_out1"
  even_adder_blk1/1 -> out_even/1  "even_delay_in2"
  sync_delay1/1 -> sync_out/1

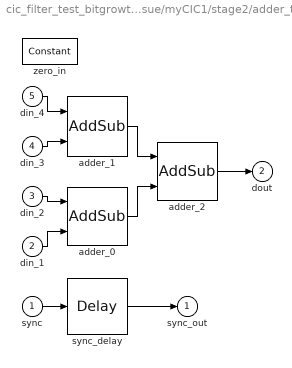
== system cic_filter_test_bitgrowthissue/myCIC1/stage2/adder_tree2 ==
  sync : Inport
  din_1 : Inport  Port=2
  din_2 : Inport  Port=3
  din_3 : Inport  Port=4
  din_4 : Inport  Port=5
  adder_0 : xbsIndex_r4/AddSub  mode=Addition  use_carryin=off  use_carryout=off  en=off  latency=1  precision=Full  arith_type=Unsigned  n_bits=16  bin_pt=14  quantization="Round  (unbiased: +/- Inf)"  overflow=Saturate  dbl_ovrd=off  use_behavioral_HDL=on  hw_selection=Fabric  pipelined=off  block_type=addsub
  adder_1 : xbsIndex_r4/AddSub  mode=Addition  use_carryin=off  use_carryout=off  en=off  latency=1  precision=Full  arith_type=Unsigned  n_bits=16  bin_pt=14  quantization="Round  (unbiased: +/- Inf)"  overflow=Saturate  dbl_ovrd=off  use_behavioral_HDL=on  hw_selection=Fabric  pipelined=off  block_type=addsub
  adder_2 : xbsIndex_r4/AddSub  mode=Addition  use_carryin=off  use_carryout=off  en=off  latency=1  precision=Full  arith_type=Unsigned  n_bits=16  bin_pt=14  quantization="Round  (unbiased: +/- Inf)"  overflow=Saturate  dbl_ovrd=off  use_behavioral_HDL=on  hw_selection=Fabric  pipelined=off  block_type=addsub
  sync_delay : xbsIndex_r4/Delay  en=off  latency=2  dbl_ovrd=off  reg_retiming=off  block_type=delay
      settings: block_version=11.4
  zero_in : xbsIndex_r4/Constant  arith_type=Unsigned  const=0  n_bits=18  bin_pt=17  explicit_period=off  period=1  equ=P=C  opselect=C  inp2=PCIN>>17  opr=+  inp1=P  carry=CIN  dbl_ovrd=off  block_type=constant
      settings: block_version=11.4
  sync_out : Outport
  dout : Outport  Port=2
  wires:
  adder_0/1 -> adder_2/2
  din_4/1 -> adder_1/1
  din_1/1 -> adder_0/2
  sync_delay/1 -> sync_out/1
  sync/1 -> sync_delay/1
  din_2/1 -> adder_0/1
  din_3/1 -> adder_1/2
  adder_1/1 -> adder_2/1
  adder_2/1 -> dout/1

== system cic_filter_test_bitgrowthissue/myCIC1/stage2/adder_tree4 ==
  sync : Inport
  din_1 : Inport  Port=2
  din_2 : Inport  Port=3
  din_3 : Inport  Port=4
  din_4 : Inport  Port=5
  adder_0 : xbsIndex_r4/AddSub  mode=Addition  use_carryin=off  use_carryout=off  en=off  latency=1  precision=Full  arith_type=Unsigned  n_bits=16  bin_pt=14  quantization="Round  (unbiased: +/- Inf)"  overflow=Saturate  dbl_ovrd=off  use_behavioral_HDL=on  hw_selection=Fabric  pipelined=off  block_type=addsub
  adder_1 : xbsIndex_r4/AddSub  mode=Addition  use_carryin=off  use_carryout=off  en=off  latency=1  precision=Full  arith_type=Unsigned  n_bits=16  bin_pt=14  quantization="Round  (unbiased: +/- Inf)"  overflow=Saturate  dbl_ovrd=off  use_behavioral_HDL=on  hw_selection=Fabric  pipelined=off  block_type=addsub
  adder_2 : xbsIndex_r4/AddSub  mode=Addition  use_carryin=off  use_carryout=off  en=off  latency=1  precision=Full  arith_type=Unsigned  n_bits=16  bin_pt=14  quantization="Round  (unbiased: +/- Inf)"  overflow=Saturate  dbl_ovrd=off  use_behavioral_HDL=on  hw_selection=Fabric  pipelined=off  block_type=addsub
  sync_delay : xbsIndex_r4/Delay  en=off  latency=2  dbl_ovrd=off  reg_retiming=off  block_type=delay
      settings: block_version=11.4
  zero_in : xbsIndex_r4/Constant  arith_type=Unsigned  const=0  n_bits=18  bin_pt=17  explicit_period=off  period=1  equ=P=C  opselect=C  inp2=PCIN>>17  opr=+  inp1=P  carry=CIN  dbl_ovrd=off  block_type=constant
      settings: block_version=11.4
  sync_out : Outport
  dout : Outport  Port=2
  wires:
  adder_0/1 -> adder_2/2
  din_4/1 -> adder_1/1
  din_1/1 -> adder_0/2
  sync_delay/1 -> sync_out/1
  sync/1 -> sync_delay/1
  din_2/1 -> adder_0/1
  din_3/1 -> adder_1/2
  adder_1/1 -> adder_2/1
  adder_2/1 -> dout/1

== system cic_filter_test_bitgrowthissue/myCIC1/stage2_/adder_tree1 ==
  sync : Inport
  din_1 : Inport  Port=2
  din_2 : Inport  Port=3
  adder_0 : xbsIndex_r4/AddSub  mode=Addition  use_carryin=off  use_carryout=off  en=off  latency=1  precision=Full  arith_type=Unsigned  n_bits=16  bin_pt=14  quantization="Round  (unbiased: +/- Inf)"  overflow=Saturate  dbl_ovrd=off  use_behavioral_HDL=on  hw_selection=Fabric  pipelined=off  block_type=addsub
  sync_delay : xbsIndex_r4/Delay  en=off  latency=1  dbl_ovrd=off  reg_retiming=off  block_type=delay
      settings: block_version=11.4
  zero_in : xbsIndex_r4/Constant  arith_type=Unsigned  const=0  n_bits=18  bin_pt=17  explicit_period=off  period=1  equ=P=C  opselect=C  inp2=PCIN>>17  opr=+  inp1=P  carry=CIN  dbl_ovrd=off  block_type=constant
      settings: block_version=11.4
  sync_out : Outport
  dout : Outport  Port=2
  wires:
  din_1/1 -> adder_0/2
  sync_delay/1 -> sync_out/1
  sync/1 -> sync_delay/1
  din_2/1 -> adder_0/1
  adder_0/1 -> dout/1

== system cic_filter_test_bitgrowthissue/myCIC1/stage2_/adder_tree2 ==
  sync : Inport
  din_1 : Inport  Port=2
  din_2 : Inport  Port=3
  adder_0 : xbsIndex_r4/AddSub  mode=Addition  use_carryin=off  use_carryout=off  en=off  latency=1  precision=Full  arith_type=Unsigned  n_bits=16  bin_pt=14  quantization="Round  (unbiased: +/- Inf)"  overflow=Saturate  dbl_ovrd=off  use_behavioral_HDL=on  hw_selection=Fabric  pipelined=off  block_type=addsub
  sync_delay : xbsIndex_r4/Delay  en=off  latency=1  dbl_ovrd=off  reg_retiming=off  block_type=delay
      settings: block_version=11.4
  zero_in : xbsIndex_r4/Constant  arith_type=Unsigned  const=0  n_bits=18  bin_pt=17  explicit_period=off  period=1  equ=P=C  opselect=C  inp2=PCIN>>17  opr=+  inp1=P  carry=CIN  dbl_ovrd=off  block_type=constant
      settings: block_version=11.4
  sync_out : Outport
  dout : Outport  Port=2
  wires:
  din_1/1 -> adder_0/2
  sync_delay/1 -> sync_out/1
  sync/1 -> sync_delay/1
  din_2/1 -> adder_0/1
  adder_0/1 -> dout/1

== system cic_filter_test_bitgrowthissue/myCIC3/stage2/adder_tree2 ==
  sync : Inport
  din_1 : Inport  Port=2
  din_2 : Inport  Port=3
  din_3 : Inport  Port=4
  din_4 : Inport  Port=5
  adder_0 : xbsIndex_r4/AddSub  mode=Addition  use_carryin=off  use_carryout=off  en=off  latency=1  precision=Full  arith_type=Unsigned  n_bits=16  bin_pt=14  quantization="Round  (unbiased: +/- Inf)"  overflow=Saturate  dbl_ovrd=off  use_behavioral_HDL=on  hw_selection=Fabric  pipelined=off  block_type=addsub
  adder_1 : xbsIndex_r4/AddSub  mode=Addition  use_carryin=off  use_carryout=off  en=off  latency=1  precision=Full  arith_type=Unsigned  n_bits=16  bin_pt=14  quantization="Round  (unbiased: +/- Inf)"  overflow=Saturate  dbl_ovrd=off  use_behavioral_HDL=on  hw_selection=Fabric  pipelined=off  block_type=addsub
  adder_2 : xbsIndex_r4/AddSub  mode=Addition  use_carryin=off  use_carryout=off  en=off  latency=1  precision=Full  arith_type=Unsigned  n_bits=16  bin_pt=14  quantization="Round  (unbiased: +/- Inf)"  overflow=Saturate  dbl_ovrd=off  use_behavioral_HDL=on  hw_selection=Fabric  pipelined=off  block_type=addsub
  sync_delay : xbsIndex_r4/Delay  en=off  latency=2  dbl_ovrd=off  reg_retiming=off  block_type=delay
      settings: block_version=11.4
  zero_in : xbsIndex_r4/Constant  arith_type=Unsigned  const=0  n_bits=18  bin_pt=17  explicit_period=off  period=1  equ=P=C  opselect=C  inp2=PCIN>>17  opr=+  inp1=P  carry=CIN  dbl_ovrd=off  block_type=constant
      settings: block_version=11.4
  sync_out : Outport
  dout : Outport  Port=2
  wires:
  adder_0/1 -> adder_2/2
  din_4/1 -> adder_1/1
  din_1/1 -> adder_0/2
  sync_delay/1 -> sync_out/1
  sync/1 -> sync_delay/1
  din_2/1 -> adder_0/1
  din_3/1 -> adder_1/2
  adder_1/1 -> adder_2/1
  adder_2/1 -> dout/1

== system cic_filter_test_bitgrowthissue/myCIC3/stage2/adder_tree4 ==
  sync : Inport
  din_1 : Inport  Port=2
  din_2 : Inport  Port=3
  din_3 : Inport  Port=4
  din_4 : Inport  Port=5
  adder_0 : xbsIndex_r4/AddSub  mode=Addition  use_carryin=off  use_carryout=off  en=off  latency=1  precision=Full  arith_type=Unsigned  n_bits=16  bin_pt=14  quantization="Round  (unbiased: +/- Inf)"  overflow=Saturate  dbl_ovrd=off  use_behavioral_HDL=on  hw_selection=Fabric  pipelined=off  block_type=addsub
  adder_1 : xbsIndex_r4/AddSub  mode=Addition  use_carryin=off  use_carryout=off  en=off  latency=1  precision=Full  arith_type=Unsigned  n_bits=16  bin_pt=14  quantization="Round  (unbiased: +/- Inf)"  overflow=Saturate  dbl_ovrd=off  use_behavioral_HDL=on  hw_selection=Fabric  pipelined=off  block_type=addsub
  adder_2 : xbsIndex_r4/AddSub  mode=Addition  use_carryin=off  use_carryout=off  en=off  latency=1  precision=Full  arith_type=Unsigned  n_bits=16  bin_pt=14  quantization="Round  (unbiased: +/- Inf)"  overflow=Saturate  dbl_ovrd=off  use_behavioral_HDL=on  hw_selection=Fabric  pipelined=off  block_type=addsub
  sync_delay : xbsIndex_r4/Delay  en=off  latency=2  dbl_ovrd=off  reg_retiming=off  block_type=delay
      settings: block_version=11.4
  zero_in : xbsIndex_r4/Constant  arith_type=Unsigned  const=0  n_bits=18  bin_pt=17  explicit_period=off  period=1  equ=P=C  opselect=C  inp2=PCIN>>17  opr=+  inp1=P  carry=CIN  dbl_ovrd=off  block_type=constant
      settings: block_version=11.4
  sync_out : Outport
  dout : Outport  Port=2
  wires:
  adder_0/1 -> adder_2/2
  din_4/1 -> adder_1/1
  din_1/1 -> adder_0/2
  sync_delay/1 -> sync_out/1
  sync/1 -> sync_delay/1
  din_2/1 -> adder_0/1
  din_3/1 -> adder_1/2
  adder_1/1 -> adder_2/1
  adder_2/1 -> dout/1

== system cic_filter_test_bitgrowthissue/myCIC3/stage2_/adder_tree1 ==
  sync : Inport
  din_1 : Inport  Port=2
  din_2 : Inport  Port=3
  adder_0 : xbsIndex_r4/AddSub  mode=Addition  use_carryin=off  use_carryout=off  en=off  latency=1  precision=Full  arith_type=Unsigned  n_bits=16  bin_pt=14  quantization="Round  (unbiased: +/- Inf)"  overflow=Saturate  dbl_ovrd=off  use_behavioral_HDL=on  hw_selection=Fabric  pipelined=off  block_type=addsub
  sync_delay : xbsIndex_r4/Delay  en=off  latency=1  dbl_ovrd=off  reg_retiming=off  block_type=delay
      settings: block_version=11.4
  zero_in : xbsIndex_r4/Constant  arith_type=Unsigned  const=0  n_bits=18  bin_pt=17  explicit_period=off  period=1  equ=P=C  opselect=C  inp2=PCIN>>17  opr=+  inp1=P  carry=CIN  dbl_ovrd=off  block_type=constant
      settings: block_version=11.4
  sync_out : Outport
  dout : Outport  Port=2
  wires:
  din_1/1 -> adder_0/2
  sync_delay/1 -> sync_out/1
  sync/1 -> sync_delay/1
  din_2/1 -> adder_0/1
  adder_0/1 -> dout/1

== system cic_filter_test_bitgrowthissue/myCIC3/stage2_/adder_tree2 ==
  sync : Inport
  din_1 : Inport  Port=2
  din_2 : Inport  Port=3
  adder_0 : xbsIndex_r4/AddSub  mode=Addition  use_carryin=off  use_carryout=off  en=off  latency=1  precision=Full  arith_type=Unsigned  n_bits=16  bin_pt=14  quantization="Round  (unbiased: +/- Inf)"  overflow=Saturate  dbl_ovrd=off  use_behavioral_HDL=on  hw_selection=Fabric  pipelined=off  block_type=addsub
  sync_delay : xbsIndex_r4/Delay  en=off  latency=1  dbl_ovrd=off  reg_retiming=off  block_type=delay
      settings: block_version=11.4
  zero_in : xbsIndex_r4/Constant  arith_type=Unsigned  const=0  n_bits=18  bin_pt=17  explicit_period=off  period=1  equ=P=C  opselect=C  inp2=PCIN>>17  opr=+  inp1=P  carry=CIN  dbl_ovrd=off  block_type=constant
      settings: block_version=11.4
  sync_out : Outport
  dout : Outport  Port=2
  wires:
  din_1/1 -> adder_0/2
  sync_delay/1 -> sync_out/1
  sync/1 -> sync_delay/1
  din_2/1 -> adder_0/1
  adder_0/1 -> dout/1

== system cic_filter_test_bitgrowthissue/non parallel CIC/stage1/polynomial0 ==
  in : Inport
  sync : Inport  Port=2
  adder_blk1 : xbsIndex_r4/AddSub  mode=Addition  use_carryin=off  use_carryout=off  en=off  latency=1  precision=Full  arith_type=Unsigned  n_bits=16  bin_pt=14  quantization=Truncate  overflow=Wrap  dbl_ovrd=off  use_behavioral_HDL=off  hw_selection=Fabric  pipelined=off  block_type=addsub
  delay1 : xbsIndex_r4/Delay  en=off  latency=1  dbl_ovrd=off  reg_retiming=off  block_type=delay
      settings: block_version=11.4
  shift_mult_array : Subsystem
  sync_delay1 : xbsIndex_r4/Delay  en=off  latency=1  dbl_ovrd=off  reg_retiming=off  block_type=delay
      settings: block_version=11.4
  out : Outport
  sync_out : Outport  Port=2
  wires:
  shift_mult_array/3(sync_out) -> sync_delay1/1  "sync_mult"
  delay1/1 -> adder_blk1/1  "delay_out1"
  shift_mult_array/1(out1) -> delay1/1  "mult_out1"
  sync/1 -> shift_mult_array/2(sync)
  in/1 -> shift_mult_array/1(in)
  shift_mult_array/2(out2) -> adder_blk1/2  "mult_out2"
  adder_blk1/1 -> out/1  "delay_in2"
  sync_delay1/1 -> sync_out/1

== system cic_filter_test_bitgrowthissue/non parallel CIC/stage1/polynomial1 ==
  in : Inport
  sync : Inport  Port=2
  adder_blk1 : xbsIndex_r4/AddSub  mode=Addition  use_carryin=off  use_carryout=off  en=off  latency=1  precision=Full  arith_type=Unsigned  n_bits=16  bin_pt=14  quantization=Truncate  overflow=Wrap  dbl_ovrd=off  use_behavioral_HDL=off  hw_selection=Fabric  pipelined=off  block_type=addsub
  delay1 : xbsIndex_r4/Delay  en=off  latency=1  dbl_ovrd=off  reg_retiming=off  block_type=delay
      settings: block_version=11.4
  shift_mult_array : Subsystem
  sync_delay1 : xbsIndex_r4/Delay  en=off  latency=1  dbl_ovrd=off  reg_retiming=off  block_type=delay
      settings: block_version=11.4
  out : Outport
  sync_out : Outport  Port=2
  wires:
  shift_mult_array/3(sync_out) -> sync_delay1/1  "sync_mult"
  delay1/1 -> adder_blk1/1  "delay_out1"
  shift_mult_array/1(out1) -> delay1/1  "mult_out1"
  sync/1 -> shift_mult_array/2(sync)
  in/1 -> shift_mult_array/1(in)
  shift_mult_array/2(out2) -> adder_blk1/2  "mult_out2"
  adder_blk1/1 -> out/1  "delay_in2"
  sync_delay1/1 -> sync_out/1

== system cic_filter_test_bitgrowthissue/non parallel CIC/stage2/polynomial0 ==
  in : Inport
  sync : Inport  Port=2
  adder_blk1 : xbsIndex_r4/AddSub  mode=Addition  use_carryin=off  use_carryout=off  en=off  latency=1  precision=Full  arith_type=Unsigned  n_bits=16  bin_pt=14  quantization=Truncate  overflow=Wrap  dbl_ovrd=off  use_behavioral_HDL=off  hw_selection=Fabric  pipelined=off  block_type=addsub
  delay1 : xbsIndex_r4/Delay  en=off  latency=1  dbl_ovrd=off  reg_retiming=off  block_type=delay
      settings: block_version=11.4
  shift_mult_array : Subsystem
  sync_delay1 : xbsIndex_r4/Delay  en=off  latency=1  dbl_ovrd=off  reg_retiming=off  block_type=delay
      settings: block_version=11.4
  out : Outport
  sync_out : Outport  Port=2
  wires:
  shift_mult_array/3(sync_out) -> sync_delay1/1  "sync_mult"
  delay1/1 -> adder_blk1/1  "delay_out1"
  shift_mult_array/1(out1) -> delay1/1  "mult_out1"
  sync/1 -> shift_mult_array/2(sync)
  in/1 -> shift_mult_array/1(in)
  shift_mult_array/2(out2) -> adder_blk1/2  "mult_out2"
  adder_blk1/1 -> out/1  "delay_in2"
  sync_delay1/1 -> sync_out/1
